simulink model "bh_spring_compress_and_tension"  (R2016a)
settings: Solver=VariableStepAuto  StartTime=0.0  StopTime=20  RelTol=1e-3
libraries: fl_lib x12, nesl_utility x4
settings Model: Creator=bhorton  LastModifiedBy=bhorton
settings DataIOCC: LimitDataPoints=on
settings DebuggingCC: AllowSymbolicDim=off
settings ModelReferenceCC: PropagateSignalLabelsOutOfModel=off
settings GRTTargetCC: GeneratePreprocessorConditionals=Use local settings

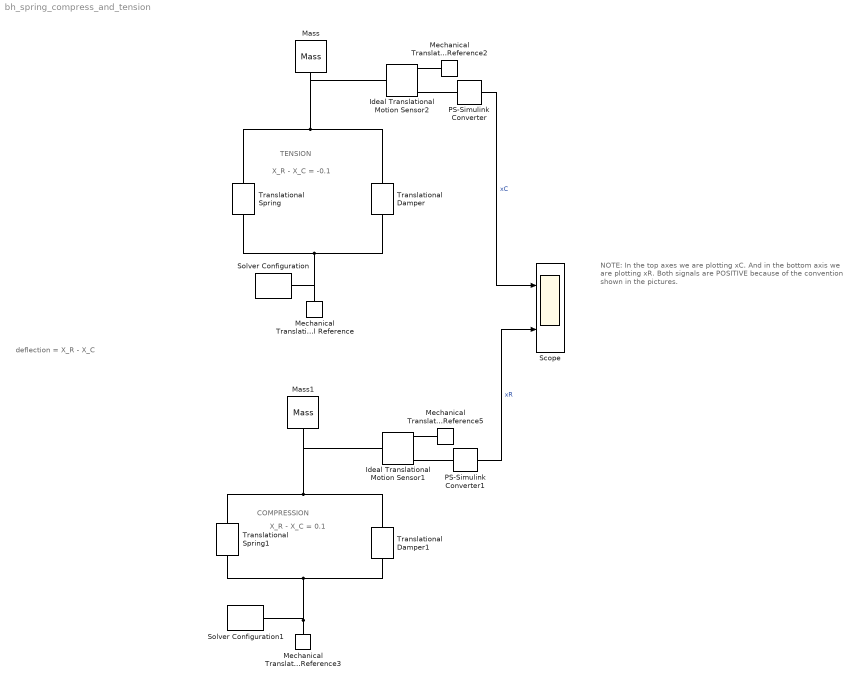
== system bh_spring_compress_and_tension ==
  note: COMPRESSION
  note: NOTE:
      | In the top axes we are plotting xC.
      | And in the bottom axis we are
      | plotting xR.
      |
      | Both signals are POSITIVE because
      | of the convention shown in the
      | pictures.
  note: X_R - X_C = 0.1
  note: deflection = X_R - X_C
  note: X_R - X_C = -0.1
  note: TENSION
  Ideal Translational Motion Sensor1 : fl_lib/Mechanical/Mechanical Sensors/Ideal Translational Motion Sensor  offset=0.1 m
      settings: AttributesFormatString=OFFSET= %<offset>
  Ideal Translational Motion Sensor2 : fl_lib/Mechanical/Mechanical Sensors/Ideal Translational Motion Sensor  offset=0.1 m
      settings: AttributesFormatString=OFFSET= %<offset>
  Mass : fl_lib/Mechanical/Translational Elements/Mass  mass=1 kg  v_specify=off  v_priority=None  v=0 m/s  f_specify=off  f_priority=None  f=0 N
  Mass1 : fl_lib/Mechanical/Translational Elements/Mass  mass=1 kg  v_specify=off  v_priority=None  v=0 m/s  f_specify=off  f_priority=None  f=0 N
  Mechanical Translational Reference{,2..3,5} (4 alike) : fl_lib/Mechanical/Translational Elements/Mechanical Translational Reference
  PS-Simulink Converter : nesl_utility/PS-Simulink Converter  PhysicalDomain=network_engine_domain  SubClassName=ps_output  LeftPortType=input  RightPortType=output  PseudoPeriodic=off  Frequencies=[]  Unit=m  AffineConversion=off
  PS-Simulink Converter1 : nesl_utility/PS-Simulink Converter  PhysicalDomain=network_engine_domain  SubClassName=ps_output  LeftPortType=input  RightPortType=output  PseudoPeriodic=off  Frequencies=[]  Unit=m  AffineConversion=off
  Scope : Scope  NumInputPorts=2
  Solver Configuration : nesl_utility/Solver Configuration  PhysicalDomain=network_engine_domain  SubClassName=solver  LeftPortType=input  RightPortType=generic  Accelerate=off  Tones=[]  Harmonics=[]  SimulateNoise=off  Profile=off  UseLocalSampling=off  EnableSwitchedLinearOptims=on  FrequencyDomain=off  UseCCode=off  RelTol=0.001  AbsTol=1e-06  MinStep=1e-09  ToWorkspace=off  RevertToSquareIcSolve=off  NumHomotopyIterations=100  PhasorMode=off  PhasorModeNumHarmonics=1  OverrideAbsTol=off  DoDC=off  ResidualTolerance=1e-09  UseLocalSolver=off  LocalSolverChoice=NE_BACKWARD_EULER_ADVANCER  LocalSolverSampleTime=0.001  DoFixedCost=off  MaxNonlinIter=3  MaxModeIter=2  LinearAlgebra=Sparse  DelaysMemoryBudget=1024  AutomaticFiltering=on  FilteringTimeConstant=0.001
  Solver Configuration1 : nesl_utility/Solver Configuration  PhysicalDomain=network_engine_domain  SubClassName=solver  LeftPortType=input  RightPortType=generic  Accelerate=off  Tones=[]  Harmonics=[]  SimulateNoise=off  Profile=off  UseLocalSampling=off  EnableSwitchedLinearOptims=on  FrequencyDomain=off  UseCCode=off  RelTol=0.001  AbsTol=1e-06  MinStep=1e-09  ToWorkspace=off  RevertToSquareIcSolve=off  NumHomotopyIterations=100  PhasorMode=off  PhasorModeNumHarmonics=1  OverrideAbsTol=off  DoDC=off  ResidualTolerance=1e-09  UseLocalSolver=off  LocalSolverChoice=NE_BACKWARD_EULER_ADVANCER  LocalSolverSampleTime=0.001  DoFixedCost=off  MaxNonlinIter=3  MaxModeIter=2  LinearAlgebra=Sparse  DelaysMemoryBudget=1024  AutomaticFiltering=on  FilteringTimeConstant=0.001
  Translational Damper : fl_lib/Mechanical/Translational Elements/Translational Damper  D=10 N/(m/s)  v_specify=off  v_priority=None  v=0 m/s  f_specify=off  f_priority=None  f=0 N
  Translational Damper1 : fl_lib/Mechanical/Translational Elements/Translational Damper  D=10 N/(m/s)  v_specify=off  v_priority=None  v=0 m/s  f_specify=off  f_priority=None  f=0 N
  Translational Spring : fl_lib/Mechanical/Translational Elements/Translational Spring  spr_rate=10 N/m  v_specify=off  v_priority=None  v=0 m/s  f_specify=off  f_priority=None  f=0 N  x_specify=on  x_priority=None  x=-0.1 m
      settings: AttributesFormatString=|
      | K=    %<spr_rate>
      | DEF=  %<x>
  Translational Spring1 : fl_lib/Mechanical/Translational Elements/Translational Spring  spr_rate=10 N/m  v_specify=off  v_priority=None  v=0 m/s  f_specify=off  f_priority=None  f=0 N  x_specify=on  x_priority=None  x=0.1 m
      settings: AttributesFormatString=|
      | K=    %<spr_rate>
      | DEF=  %<x>
  wires:
  PS-Simulink Converter/1 -> Scope/1  "xC"
  PS-Simulink Converter1/1 -> Scope/2  "xR"
  connections:
  Translational Damper/LConn1 -- Solver Configuration/RConn1 -- Mechanical Translational Reference/LConn1 -- Translational Spring/LConn1
  Translational Damper/RConn1 -- Ideal Translational Motion Sensor2/LConn1 -- Mass/LConn1 -- Translational Spring/RConn1
  Ideal Translational Motion Sensor1/RConn3 -- PS-Simulink Converter1/LConn1
  Ideal Translational Motion Sensor1/RConn1 -- Mechanical Translational Reference5/LConn1
  Translational Spring1/RConn1 -- Mechanical Translational Reference3/LConn1 -- Solver Configuration1/RConn1 -- Translational Damper1/RConn1
  Mechanical Translational Reference2/LConn1 -- Ideal Translational Motion Sensor2/RConn1
  PS-Simulink Converter/LConn1 -- Ideal Translational Motion Sensor2/RConn3
  Translational Spring1/LConn1 -- Ideal Translational Motion Sensor1/LConn1 -- Mass1/LConn1 -- Translational Damper1/LConn1
